simulink model "testScript_model"  (R2013a)
settings: Solver=ode45  SolverMode=SingleTasking  StartTime=0.0  StopTime=3000.0  RelTol=1e-3
values from neighbouring files (symbols this model uses):
  CMD_signals = [0 300 600 900 1200 1500 1800 2100 2400 2700 3000 3300 ... (1568 elements, 49x32)]    [CMD_signals.mat]
libraries: powerlib x9, powerlib_meascontrol x1
settings Model: Creator=ma25949  LastModifiedBy=ed12083
settings DataIOCC: SignalLoggingSaveFormat=ModelDataLogs
settings OptimizationCC: BlockReduction=off  BooleanDataType=off
settings DebuggingCC: SaveWithParameterizedLinksMsg=none  SignalResolutionControl=TryResolveAllWithWarning  SolverPrmCheckMsg=none  MultiTaskDSMMsg=warning  MultiTaskCondExecSysMsg=none  StrictBusMsg=None
settings HardwareCC: TargetUnknown=on
settings RTWCC: IncludeERTFirstTime=on

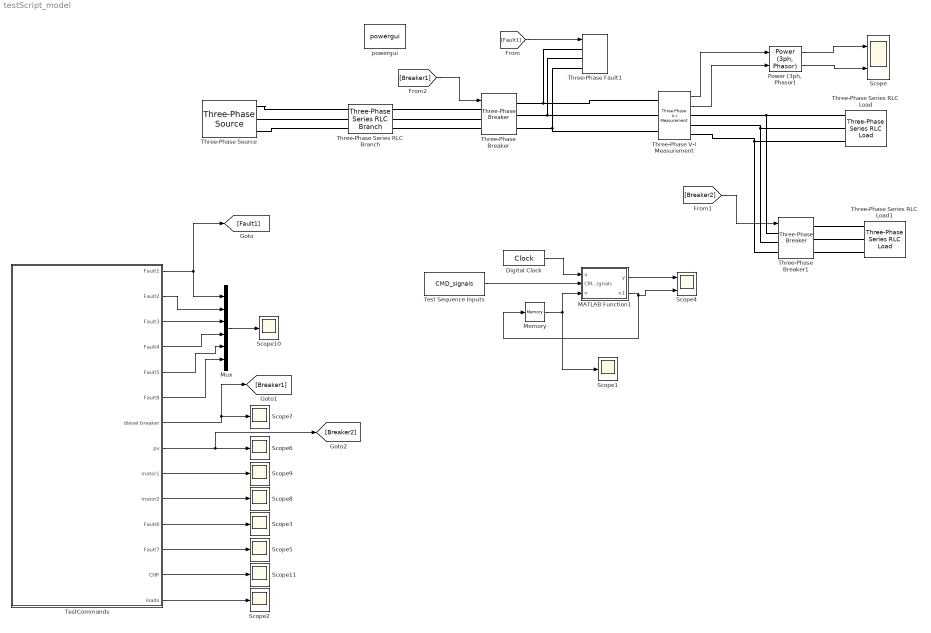
== system testScript_model ==
  Digital Clock : DigitalClock
  MATLAB Function1 : MATLAB Function  TreatAsAtomicUnit=on
  Memory : Memory  X0=1
  Mux : Mux  Inputs=6
  "Power (3ph, Phasor)" : powerlib_meascontrol/Measurements/Power (3ph, Phasor)
  Scope : Scope  NumInputPorts=2
      settings: YMin=-5~-5  YMax=5~5
  Scope{1..3,5..11} (10 alike) : Scope
      Scope10 settings: SaveName=ScopeData8
      Scope11 settings: SaveName=ScopeData11
      Scope2 settings: SaveName=ScopeData2
      Scope3 settings: SaveName=ScopeData3
      Scope5 settings: SaveName=ScopeData5
      Scope6 settings: SaveName=ScopeData6
      Scope7 settings: SaveName=ScopeData7
      Scope8 settings: SaveName=ScopeData9
      Scope9 settings: SaveName=ScopeData10
  Scope4 : Scope  NumInputPorts=3
      settings: YMin=-5~-5~-5  YMax=5~5~5  SaveName=ScopeData4
  Test Sequence Inputs : Constant  Value=CMD_signals
  TestCommands : Subsystem  mask{fault1=0, fault7=0, pv_breaker=0, fault4=0, fault8=0, fault2=0, motor1_breaker=1, fault5=0, motor2_breaker=0, fault3=0, diesel_breaker=0, fault6=0, CHP_breaker=0, load_gain=0.5}
      mask prompts: pv_breaker "PV breaker"; motor1_breaker "Motor 1 breaker"; motor2_breaker "Motor 2 breaker"; diesel_breaker "Diesel breaker"; CHP_breaker "CHP"; load_gain "Loads"
  Three-Phase Series RLC Branch : powerlib/Elements/Three-Phase Series RLC Branch  LConnTagsString=A|B|C  RConnTagsString=A|B|C  BranchType=RLC  Resistance=1  Inductance=1e-3  Capacitance=1e-6  Measurements=None
  Three-Phase Series RLC Load : powerlib/Elements/Three-Phase Series RLC Load  LConnTagsString=A|B|C  Configuration=Y (grounded)  NominalVoltage=1000  NominalFrequency=60  ActivePower=10e3  InductivePower=100  CapacitivePower=100  Measurements=None  LoadType=constant Z
  Three-Phase Series RLC Load1 : powerlib/Elements/Three-Phase Series RLC Load  LConnTagsString=A|B|C  Configuration=Y (grounded)  NominalVoltage=1000  NominalFrequency=60  ActivePower=10e3  InductivePower=100  CapacitivePower=100  Measurements=None  LoadType=constant Z
  Three-Phase V-I Measurement : powerlib/Measurements/Three-Phase V-I Measurement  VoltageMeasurement=phase-to-ground  SetLabelV=off  LabelV=Vabc  Vpu=off  VpuLL=off  CurrentMeasurement=yes  SetLabelI=off  LabelI=Iabc  Ipu=off  Pbase=100e6  Vbase=500e3  OutputType=Complex  PhasorSimulation=on  PSBequivalent=0
  Three-Phase Breaker : powerlib/Elements/Three-Phase Breaker  InitialState=closed  SwitchA=on  SwitchB=on  SwitchC=on  SwitchTimes="[15  20]"  External=on  BreakerResistance=0.001  SnubberResistance=1e6  SnubberCapacitance=inf  Measurements=Breaker voltages and currents
  Three-Phase Breaker1 : powerlib/Elements/Three-Phase Breaker  InitialState=closed  SwitchA=on  SwitchB=on  SwitchC=on  SwitchTimes="[15  20]"  External=on  BreakerResistance=0.001  SnubberResistance=1e6  SnubberCapacitance=inf  Measurements=Breaker voltages and currents
  Three-Phase Fault1 : powerlib/Elements/Three-Phase Fault  FaultA=on  FaultB=on  FaultC=on  FaultResistance=0.001  GroundFault=on  GroundResistance=100  External=on  SwitchStatus=[1 0]  SwitchTimes=[ 1/60 5/60]  InitialStates=[0 0 1]  SnubberResistance=1e6  SnubberCapacitance=inf  Measurements=None
  Three-Phase Source : powerlib/Electrical Sources/Three-Phase Source  Voltage=25e3  PhaseAngle=0  Frequency=60  InternalConnection=Yg  SpecifyImpedance=on  Resistance=0.8929  Inductance=16.58e-3  ShortCircuitLevel=100e6  BaseVoltage=25e3  XRratio=7  BusType=swing  Pref=0  Qref=0  Qmin=-inf  Qmax=inf
  powergui : powerlib/powergui  Priority=1  SimulationMode=Phasor  SolverType=Tustin  SampleTime=50e-6  frequency=60  SPID=off  DisableSnubberDevices=off  DisableRonSwitches=off  DisableVfSwitches=off  SwTol=0  Interpol=off  DisplayEquations=off  frequencyindice=60  Pbase=100e6  ErrMax=1e-4  Iterations=50  UnitsV=kV  UnitsW=MW  FunctionMessages=off  echomessages=off  HookPort=off  EnableUseOfTLC=off  x0status=blocks  RestoreLinks=warning  ResistiveCurrentMeasurement=off  Frange=[0:2:500]  Ylog=off  Xlog=on  ShowGrid=off  save=off  variable=ZData  structure=0  ZoomFFT=off  StartTime=0.0  cycles=1  DisplayStyle=1  fundamental=60  FreqAxis=off  MaxFrequency=1000  frequencyindicesteady=1  RmsSteady=1  display=off  Ts=0  methode=off
  wires:
  Three-Phase V-I Measurement/2 -> "Power (3ph, Phasor)"/2
  Three-Phase V-I Measurement/1 -> "Power (3ph, Phasor)"/1
  "Power (3ph, Phasor)"/1 -> Scope/1
  "Power (3ph, Phasor)"/2 -> Scope/2
  Digital Clock/1 -> MATLAB Function1/1(u)
  MATLAB Function1/1(y) -> Scope4/1
  [Fault1] -> Three-Phase Fault1/1
  [Breaker2] -> Three-Phase Breaker1/1
  [Breaker1] -> Three-Phase Breaker/1
  TestCommands/1(Fault1) -> Mux/1, [Fault1]
  TestCommands/2(Fault2) -> Mux/2
  TestCommands/3(Fault3) -> Mux/3
  TestCommands/4(Fault4) -> Mux/4
  TestCommands/5(Fault5) -> Mux/5
  TestCommands/6("Fault8 ") -> Mux/6
  Mux/1 -> Scope10/1
  TestCommands/7(diesel breaker) -> [Breaker1], Scope7/1
  TestCommands/8(pv) -> [Breaker2], Scope6/1
  MATLAB Function1/2(n1) -> Scope4/3, Memory/1
  Memory/1 -> Scope1/1, MATLAB Function1/3(n)
  Test Sequence Inputs/1 -> MATLAB Function1/2(CMD_signals)
  TestCommands/14(loads) -> Scope2/1
  TestCommands/11(Fault6) -> Scope3/1
  TestCommands/12(Fault7) -> Scope5/1
  TestCommands/13(CHP) -> Scope11/1
  TestCommands/9(motor1) -> Scope9/1
  TestCommands/10(motor2) -> Scope8/1
  connections:
  Three-Phase Source/RConn1 -- Three-Phase Series RLC Branch/LConn1
  Three-Phase Source/RConn2 -- Three-Phase Series RLC Branch/LConn2
  Three-Phase Source/RConn3 -- Three-Phase Series RLC Branch/LConn3
  Three-Phase Series RLC Branch/RConn2 -- Three-Phase Breaker/LConn2
  Three-Phase Breaker/RConn2 -- Three-Phase Fault1/LConn2 -- Three-Phase V-I Measurement/LConn2
  Three-Phase Breaker/RConn3 -- Three-Phase Fault1/LConn3 -- Three-Phase V-I Measurement/LConn3
  Three-Phase Breaker/RConn1 -- Three-Phase Fault1/LConn1 -- Three-Phase V-I Measurement/LConn1
  Three-Phase V-I Measurement/RConn2 -- Three-Phase Breaker1/LConn2 -- Three-Phase Series RLC Load/LConn2
  Three-Phase V-I Measurement/RConn3 -- Three-Phase Breaker1/LConn3 -- Three-Phase Series RLC Load/LConn3
  Three-Phase V-I Measurement/RConn1 -- Three-Phase Breaker1/LConn1 -- Three-Phase Series RLC Load/LConn1
  Three-Phase Series RLC Branch/RConn1 -- Three-Phase Breaker/LConn1
  Three-Phase Series RLC Branch/RConn3 -- Three-Phase Breaker/LConn3
  Three-Phase Breaker1/RConn1 -- Three-Phase Series RLC Load1/LConn1
  Three-Phase Breaker1/RConn2 -- Three-Phase Series RLC Load1/LConn2
  Three-Phase Breaker1/RConn3 -- Three-Phase Series RLC Load1/LConn3

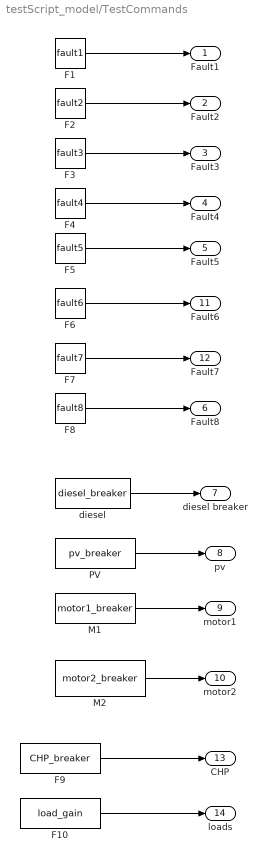
== system testScript_model/TestCommands ==
  F1 : Constant  Value=fault1
  F10 : Constant  Value=load_gain
  F2 : Constant  Value=fault2
  F3 : Constant  Value=fault3
  F4 : Constant  Value=fault4
  F5 : Constant  Value=fault5
  F6 : Constant  Value=fault6
  F7 : Constant  Value=fault7
  F8 : Constant  Value=fault8
  F9 : Constant  Value=CHP_breaker
  M1 : Constant  Value=motor1_breaker
  M2 : Constant  Value=motor2_breaker
  PV : Constant  Value=pv_breaker
  diesel : Constant  Value=diesel_breaker
  Fault1 : Outport
  Fault2 : Outport  Port=2
  Fault3 : Outport  Port=3
  Fault4 : Outport  Port=4
  Fault5 : Outport  Port=5
  "Fault8 " : Outport  Port=6
  diesel breaker : Outport  Port=7
  pv : Outport  Port=8
  motor1 : Outport  Port=9
  motor2 : Outport  Port=10
  Fault6 : Outport  Port=11
  Fault7 : Outport  Port=12
  CHP : Outport  Port=13
  loads : Outport  Port=14
  wires:
  F1/1 -> Fault1/1
  F2/1 -> Fault2/1
  F3/1 -> Fault3/1
  F4/1 -> Fault4/1
  F5/1 -> Fault5/1
  F8/1 -> "Fault8 "/1
  diesel/1 -> diesel breaker/1
  PV/1 -> pv/1
  M1/1 -> motor1/1
  M2/1 -> motor2/1
  F6/1 -> Fault6/1
  F7/1 -> Fault7/1
  F9/1 -> CHP/1
  F10/1 -> loads/1

== matlab function testScript_model/MATLAB Function1 ==
  data: u input; y output; CMD_signals input; n input; n1 output
function [y,n1] = fcn(u,CMD_signals,n)
% Author: Matthew Backes, MIT Lincoln Laboratory
% Date: 8/16/2016
% This function takes in the test sequence signals from a .mat file which
% is generated with the ____.m script. It then updates the parameters
% within the simulink model according to the time stamp of the test
% sequence command signals.
% CMD column 1 = time
% CMD column 2 = POI feeder 1 SEL relay
% CMD column 3 = POI feeder 2 SEL relay
% CMD column 4 = POI feeder 3 SEL relay
% CMD column 5 = diesel breaker
% CMD column 6 = solar irradiance gain
% CMD column 7 = solar breaker
% CMD column 8 = CHP breaker
% CMD column 9 = load gain
% CMD column 10 = motor 1 breaker
% CMD column 11 = motor 2 breaker
% CMD column 12 = fault location 1
% CMD column 13 = fault location 2
% CMD column 14 = fault location 3
% CMD column 15 = fault location 4
% CMD column 16 = fault location 5
% CMD column 17 = fault location 6
% CMD column 18 = fault location 7
% CMD column 19 = fault location 8
% CMD column 20 = dso Disconnect command
% CMD column 21 = dso Reconnect command
% CMD column 22 = dso Export command
% CMD column 23 = dso Import command
% CMD column 24 = dso power factor command
% CMD column 25 = dso VAR support command
% CMD column 26 = dso Demand Response command
% CMD column 27 = dso Import/export value
% CMD column 28 = dso power factor value
% CMD column 29 = dso VAR value
% CMD column 30 = dso DR value
% CMD column 31 = dso Command start time
% CMD column 32 = dso command duration

y = u;

coder.extrinsic('set_param') %declare set_param as an extrinsic function
coder.extrinsic('num2str') %declare num2str as an extrinsic function
coder.extrinsic('tcpip')

time = CMD_signals(:,1); 
%time_lastCMD = time(length(time)); %do i need this anymore?
numCMDs = length(time);
DMS_ipaddr = '192.168.10.40';
POI_F1_ipaddr = '192.168.10.41';
POI_F2_ipaddr = '192.168.10.42';
POI_F3_ipaddr = '192.168.10.43';
port = 512;

handles.tcp=tcpip(DMS_ipaddr, port,'Timeout',1);    %Create the tcpip object
set(handles.tcp, 'InputBufferSize', 512);       %assign the buffer
handles.tcp.ByteOrder='bigEndian';              %specify the order in which bytes are transmitted

handles.connected=0;                            %default is not connected
% try 
    if ~strcmp(handles.tcp.Status,'open')       %if not open then 
        fopen(handles.tcp);                     %open a connection
        handles.connected = 1;                  %connected
    end


if n > numCMDs   %do nothing if we have exhausted all commands
    n1 = n;
else
    if u > time(n) % when the simulation time is greater than the command signal time, execute set_param
        n1 = n+1; % increment to next command to execute
        
        %parameters to set within simulink model
        set_param('testScript_model/TestCommands','diesel_breaker',num2str(CMD_signals(n,5)),'pv_breaker',num2str(CMD_signals(n,7)),'CHP_breaker',num2str(CMD_signals(n,8)),'load_gain',num2str(CMD_signals(n,9)),'motor1_breaker',num2str(CMD_signals(n,10)),'motor2_breaker',num2str(CMD_signals(n,11)),'fault1',num2str(CMD_signals(n,12)),'fault2',num2str(CMD_signals(n,13)),'fault3',num2str(CMD_signals(n,14)),'fault4',num2str(CMD_signals(n,15)),'fault5',num2str(CMD_signals(n,16)),'fault6',num2str(CMD_signals(n,17)),'fault7',num2str(CMD_signals(n,18)),'fault8',num2str(CMD_signals(n,19)));
        
        %modbus commands
%         if CMD_signals(n,2) == 1    %if 1, then POI_1 should be open -> issue Modbus command
%             ctrl_device_DMS_modbus(POI_F1_ipaddr,502,[20,0,6,1,6,hex2dec('2000'),2]);
%         else
%             ctrl_device_DMS_modbus(POI_F1_ipaddr,502,[20,0,6,1,6,hex2dec('2001'),1]);
%         end
%         if CMD_signals(n,3) == 1
%             ctrl_device_DMS_modbus(POI_F2_ipaddr,502,[20,0, 6, 1, 6, 2000, 2]);
%         else
%             ctrl_device_DMS_modbus(POI_F2_ipaddr,502,[20,0,6,1,6,2001,1]);
%         end
%         if CMD_signals(n,4) == 1
%             ctrl_device_DMS_modbus(POI_F3_ipaddr,502,[20,0,6,1,6,2000,2]);
%         else
%             ctrl_device_DMS_modbus(POI_F3_ipaddr,502,[20,0,6,1,6,2001,1]);
%         end
%         
%         if dsoDisconnect(n) == 1 
%             ctrl_device_DMS_modbus(DMS_ipaddr,502,[10, 0, 6, 1, 6, 0000, 1]); %do i need to reset this?
%         end
%         if dsoReconnect(n) == 1 
%             ctrl_device_DMS_modbus(DMS_ipaddr,502,[10, 0, 6, 1, 6, 0001, 1]);
%         end
%         if dsoExport(n) == 1
%             ctrl_device_DMS_modbus(DMS_ipaddr,502,[10, 0, 6, 1, 6, 0002, 1]);
%             ctrl_device_DMS_modbus(DMS_ipaddr,502,[10, 0, 6, 1, 6, 0007, CMD_Signals(n,27)]);
%         end
%         if dsoImport(n) == 1
%             ctrl_device_DMS_modbus(DMS_ipaddr,502,[10, 0, 6, 1, 6, 0003, 1]);
%             ctrl_device_DMS_modbus(DMS_ipaddr,502,[10, 0, 6, 1, 6, 0007, CMD_Signals(n,27)]);
%         end
%         if dsoPF(n) == 1 
%             ctrl_device_DMS_modbus(DMS_ipaddr,502,[10, 0, 6, 1, 6, 0004, 1]);
%             ctrl_device_DMS_modbus(DMS_ipaddr,502,[10, 0, 6, 1, 6, 0008, CMD_Signals(n,28)]);
%         end
%         if dsoVAR(n) == 1
%             ctrl_device_DMS_modbus(DMS_ipaddr,502,[10, 0, 6, 1, 6, 0005, 1]);
%             ctrl_device_DMS_modbus(DMS_ipaddr,502,[10, 0, 6, 1, 6, 0009, CMD_Signals(n,29)]);
%         end
%         if dsoDR(n) == 1
%             ctrl_device_DMS_modbus(DMS_ipaddr,502,[10, 0, 6, 1, 6, 0006, 1]);
%             ctrl_device_DMS_modbus(DMS_ipaddr,502,[10, 0, 6, 1, 6, 0010, CMD_Signals(n,30)]);
%         end
%         
%         ctrl_device_DMS_modbus(DMS_ipaddr,502,[10, 0, 6, 1, 6, 0011, u]);
%         ctrl_device_DMS_modbus(DMS_ipaddr,502,[10, 0, 6, 1, 6, 0012, CMD_Signals(n,31)]);
%         ctrl_device_DMS_modbus(DMS_ipaddr,502,[10, 0, 6, 1, 6, 0013, CMD_Signals(n,32)]);
        
     else  % wait until the simulation time has eclisped the next command time
        n1 = n; 
    end
end
